simulink library "lib_decmp_CtrSet_tbm_enab_x8"  (R2020a)
settings: Solver=VariableStepAuto  StartTime=0.0  StopTime=10.0  RelTol=1e-3
settings Model: Creator=Administrator  LastModifiedBy=Administrator

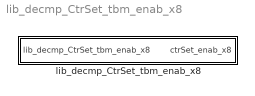
== system lib_decmp_CtrSet_tbm_enab_x8 ==
  lib_decmp_CtrSet_tbm_enab_x8 : Subsystem

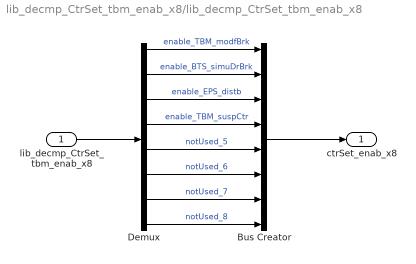
== system lib_decmp_CtrSet_tbm_enab_x8/lib_decmp_CtrSet_tbm_enab_x8 ==
  lib_decmp_CtrSet_tbm_enab_x8 : Inport  OutDataTypeStr=boolean  PortDimensions=8
  Bus Creator : BusCreator  Inputs=8
  Demux : Demux  Outputs=8
  ctrSet_enab_x8 : Outport  PortDimensions=8
  wires:
  lib_decmp_CtrSet_tbm_enab_x8/1 -> Demux/1
  Demux/1 -> Bus Creator/1  "enable_TBM_modfBrk"
  Demux/2 -> Bus Creator/2  "enable_BTS_simuDrBrk"
  Demux/3 -> Bus Creator/3  "enable_EPS_distb"
  Demux/4 -> Bus Creator/4  "enable_TBM_suspCtr"
  Bus Creator/1 -> ctrSet_enab_x8/1
  Demux/5 -> Bus Creator/5  "notUsed_5"
  Demux/6 -> Bus Creator/6  "notUsed_6"
  Demux/7 -> Bus Creator/7  "notUsed_7"
  Demux/8 -> Bus Creator/8  "notUsed_8"
